simulink model "two_segment_model"  (R2024b)
settings: Solver=VariableStepAuto  StartTime=0.0  StopTime=0.64  MaxStep=0.001  RelTol=1e-6
values from neighbouring files (symbols this model uses):
  attack_angle = 90    [params.m]
  c = log(0.05)    [params.m]
  d = 0.04    [params.m]
  delP = 0.015    [params.m]
  e_ref_see = 0.04    [params.m]
  F_max = 22000    [params.m]
  g = 9.81    [params.m]
  G = 1.84/F_max    (= 8.36363636364e-05)    [params.m]
  K = 5    [params.m]
  l_f = 0.99    [params.m]
  l_off = 0.08    [params.m]
  l_opt = 0.1    [params.m]
  l_ref_mtc = 0.5    [params.m]
  l_rest = 0.4    [params.m]
  l_s = 0.5    [params.m]
  m = 80    [params.m]
  N = 1.5    [params.m]
  phi_initial = 2*rad2deg(atan(l_f/(2*sqrt(l_s^2 - l_f^2/4))))    [params.m]
  phi_ref_mtc = 110    [params.m]
  stim0 = 0.145    [params.m]
  tau = 0.01    [params.m]
  v_max = 12*l_opt    (= 1.2)    [params.m]
  w = 0.4    [params.m]
libraries: simulink_extras x1
settings Model: Creator=athar  LastModifiedBy=athar

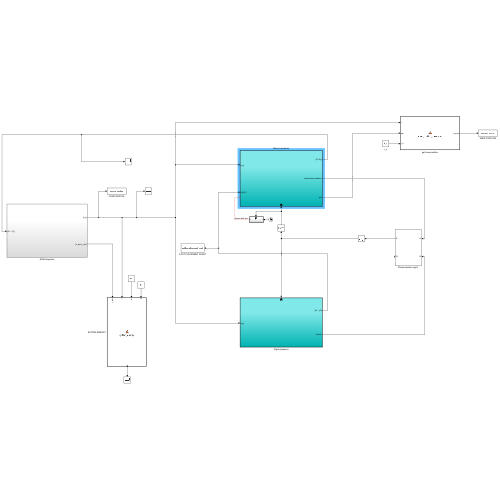
[thumbnail: Simulink's stored preview of the top-level diagram]
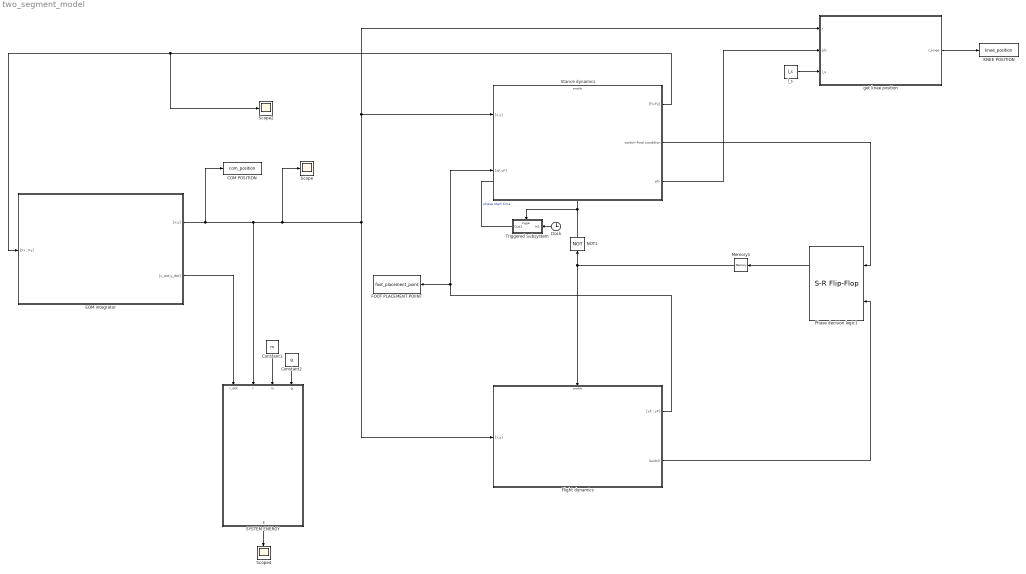
== system two_segment_model ==
  COM POSITION : ToWorkspace  VariableName=com_position  SampleTime=-1
      settings: Save2DSignal=2-D array (concatenate along first dimension)
  Clock : Clock
  Constant1 : Constant  Value=m
  Constant2 : Constant  Value=g
  EOM integrator : Subsystem
  FOOT PLACEMENT POIINT : ToWorkspace  VariableName=foot_placement_point  SampleTime=-1
      settings: Save2DSignal=2-D array (concatenate along first dimension)
  Flight dynamics : Subsystem
  KNEE POSITION : ToWorkspace  VariableName=knee_position  SampleTime=-1
      settings: Save2DSignal=2-D array (concatenate along first dimension)
  Memory1 : Memory  InitialCondition=1
  NOT1 : Logic  Operator=NOT  AllPortsSameDT=off  OutDataTypeStr=boolean
  Phase decision logic1 : simulink_extras/Flip Flops/S-R Flip-Flop  initial_condition=1
  SYSTEM ENERGY : MATLAB Function  TreatAsAtomicUnit=on
  Scope : Scope
  Scope2 : Scope
  Scope4 : Scope
  Stance dynamics : Subsystem
  Triggered Subsystem : Subsystem  TreatAsAtomicUnit=on
  get knee position : MATLAB Function  TreatAsAtomicUnit=on
  l_s : Constant  Value=l_s
  wires:
  Flight dynamics/1("[xF ; yF]") -> Stance dynamics/2("[xF,yF]"), FOOT PLACEMENT POIINT/1
  Stance dynamics/1("[Fx;Fy]") -> Scope2/1, EOM integrator/1("[Fx ; Fy]")
  Memory1/1 -> NOT1/1, Flight dynamics/Enable
  Flight dynamics/2(Switch) -> Phase decision logic1/2
  Phase decision logic1/1 -> Memory1/1
  NOT1/1 -> Triggered Subsystem/Trigger, Stance dynamics/Enable
  Stance dynamics/2(switch-final condition) -> Phase decision logic1/1
  EOM integrator/2("[x_dot;y_dot]") -> SYSTEM ENERGY/1(r_dot)
  Constant1/1 -> SYSTEM ENERGY/3(m)
  Constant2/1 -> SYSTEM ENERGY/4(g)
  SYSTEM ENERGY/1(E) -> Scope4/1
  Clock/1 -> Triggered Subsystem/1(In1)
  Triggered Subsystem/1(Out1) -> ?  "phase start time"
  EOM integrator/1("[x;y]") -> COM POSITION/1, SYSTEM ENERGY/2(r), Scope/1, Flight dynamics/1("[x;y]"), get knee position/1(r), Stance dynamics/1("[x,y]")
  Stance dynamics/3(phi) -> get knee position/2(phi)
  l_s/1 -> get knee position/3(l_s)
  get knee position/1(r_knee) -> KNEE POSITION/1

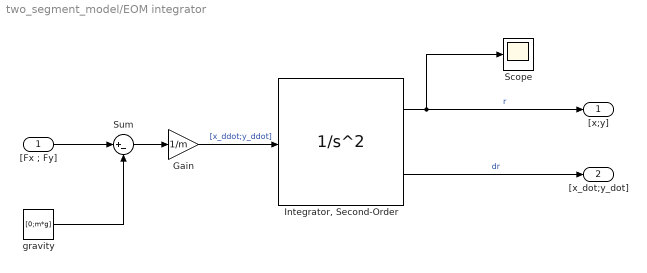
== system two_segment_model/EOM integrator ==
  "[Fx ; Fy]" : Inport
  Gain : Gain  Gain=1/m
  "Integrator, Second-Order" : SecondOrderIntegrator  ICX=r0  ICDXDT=r_dot0
  Scope : Scope
  Sum : Sum  Inputs=|+-
  gravity : Constant  Value=[0;m*g]
  "[x;y]" : Outport
  "[x_dot;y_dot]" : Outport  Port=2
  wires:
  "Integrator, Second-Order"/2 -> "[x_dot;y_dot]"/1  "dr"
  "Integrator, Second-Order"/1 -> Scope/1, "[x;y]"/1  "r"
  "[Fx ; Fy]"/1 -> Sum/1
  Sum/1 -> Gain/1
  gravity/1 -> Sum/2
  Gain/1 -> "Integrator, Second-Order"/1  "[x_ddot;y_ddot]"

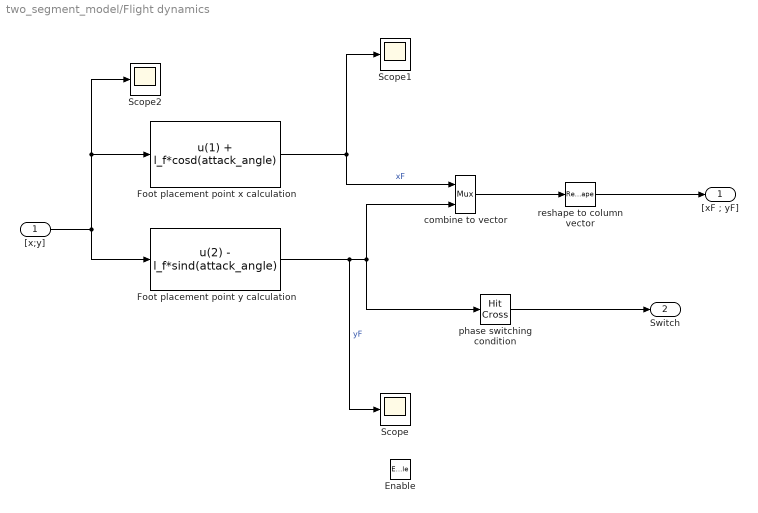
== system two_segment_model/Flight dynamics ==
  "[x;y]" : Inport
  Enable : EnablePort  StatesWhenEnabling=reset
  Foot placement point x calculation : Fcn  Expr=u(1) + l_f*cosd(attack_angle)
  Foot placement point y calculation : Fcn  Expr=u(2) - l_f*sind(attack_angle)
  Scope : Scope
  Scope1 : Scope
  Scope2 : Scope
  combine to vector : Mux  Inputs=2
  phase switching condition : HitCross  HitCrossingOffset=yG  HitCrossingDirection=falling
  reshape to column vector : Reshape  OutputDimensionality=Column vector (2-D)
  "[xF ; yF]" : Outport  InitialOutput=[0;0]
  Switch : Outport  Port=2  OutputWhenDisabled=reset  InitialOutput=0
  wires:
  "[x;y]"/1 -> Foot placement point y calculation/1, Scope2/1, Foot placement point x calculation/1
  Foot placement point y calculation/1 -> Scope/1, combine to vector/2, phase switching condition/1  "yF"
  Foot placement point x calculation/1 -> Scope1/1, combine to vector/1  "xF"
  combine to vector/1 -> reshape to column vector/1
  phase switching condition/1 -> Switch/1
  reshape to column vector/1 -> "[xF ; yF]"/1

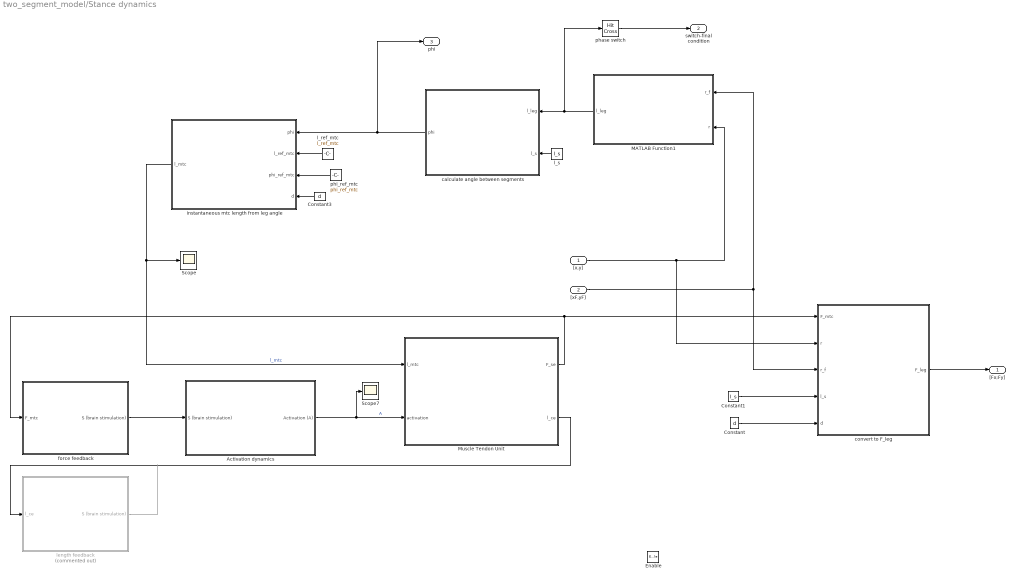
== system two_segment_model/Stance dynamics ==
  "[x,y]" : Inport
  "[xF,yF]" : Inport  Port=2
  Enable : EnablePort  StatesWhenEnabling=reset
  Activation dynamics : Subsystem
  Constant : Constant  Value=d
  Constant1 : Constant  Value=l_s
  Constant3 : Constant  Value=d
  MATLAB Function1 : MATLAB Function  TreatAsAtomicUnit=on
  Muscle Tendon Unit : Subsystem
  Scope : Scope
  Scope7 : Scope
  calculate angle between segments : MATLAB Function  TreatAsAtomicUnit=on
  convert to F_leg : MATLAB Function  TreatAsAtomicUnit=on
  force feedback : Subsystem
  instantaneous mtc length from leg angle : MATLAB Function  TreatAsAtomicUnit=on
  l_ref_mtc : Constant  Value=l_ref_mtc
  l_s : Constant  Value=l_s
  length feedback : Subsystem  Commented=on
  phase switch : HitCross  HitCrossingOffset=l_f  HitCrossingDirection=rising
  phi_ref_mtc : Constant  Value=phi_ref_mtc
  "[Fx;Fy]" : Outport  OutputWhenDisabled=reset  InitialOutput=[0;0]
  switch-final condition : Outport  Port=2  OutputWhenDisabled=reset  InitialOutput=0
  phi : Outport  Port=3  InitialOutput=phi_initial
  wires:
  "[xF,yF]"/1 -> MATLAB Function1/1(r_f), convert to F_leg/3(r_f)
  convert to F_leg/1(F_leg) -> "[Fx;Fy]"/1
  instantaneous mtc length from leg angle/1(l_mtc) -> Scope/1, Muscle Tendon Unit/1(l_mtc)  "l_mtc"
  l_ref_mtc/1 -> instantaneous mtc length from leg angle/2(l_ref_mtc)
  "[x,y]"/1 -> MATLAB Function1/2(r), convert to F_leg/2(r)
  Activation dynamics/1(Activation (A)) -> Scope7/1, Muscle Tendon Unit/2(activation)  "A"
  phi_ref_mtc/1 -> instantaneous mtc length from leg angle/3(phi_ref_mtc)
  Muscle Tendon Unit/1(F_se) -> force feedback/1(F_mtc), convert to F_leg/1(F_mtc)
  Constant/1 -> convert to F_leg/5(d)
  Constant1/1 -> convert to F_leg/4(l_s)
  l_s/1 -> calculate angle between segments/2(l_s)
  calculate angle between segments/1(phi) -> phi/1, instantaneous mtc length from leg angle/1(phi)
  Constant3/1 -> instantaneous mtc length from leg angle/4(d)
  MATLAB Function1/1(l_leg) -> phase switch/1, calculate angle between segments/1(l_leg)
  phase switch/1 -> switch-final condition/1
  Muscle Tendon Unit/2(l_ce) -> length feedback/1(l_ce)
  length feedback/1(S (brain stimulation)) -> ?
  force feedback/1(S (brain stimulation)) -> Activation dynamics/1(S (brain stimulation))

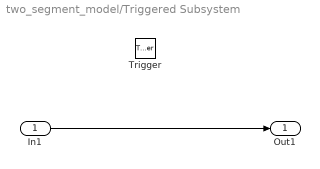
== system two_segment_model/Triggered Subsystem ==
  In1 : Inport
  Trigger : TriggerPort  VariantControl=(inherit)
  Out1 : Outport
  wires:
  In1/1 -> Out1/1

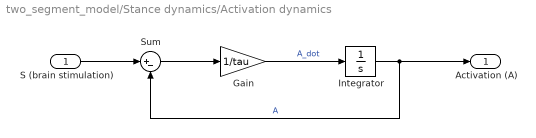
== system two_segment_model/Stance dynamics/Activation dynamics ==
  S (brain stimulation) : Inport
  Gain : Gain  Gain=1/tau
  Integrator : Integrator  InitialCondition=0.001
  Sum : Sum  Inputs=|+-
  Activation (A) : Outport
  wires:
  S (brain stimulation)/1 -> Sum/1
  Sum/1 -> Gain/1
  Gain/1 -> Integrator/1  "A_dot"
  Integrator/1 -> Sum/2, Activation (A)/1  "A"

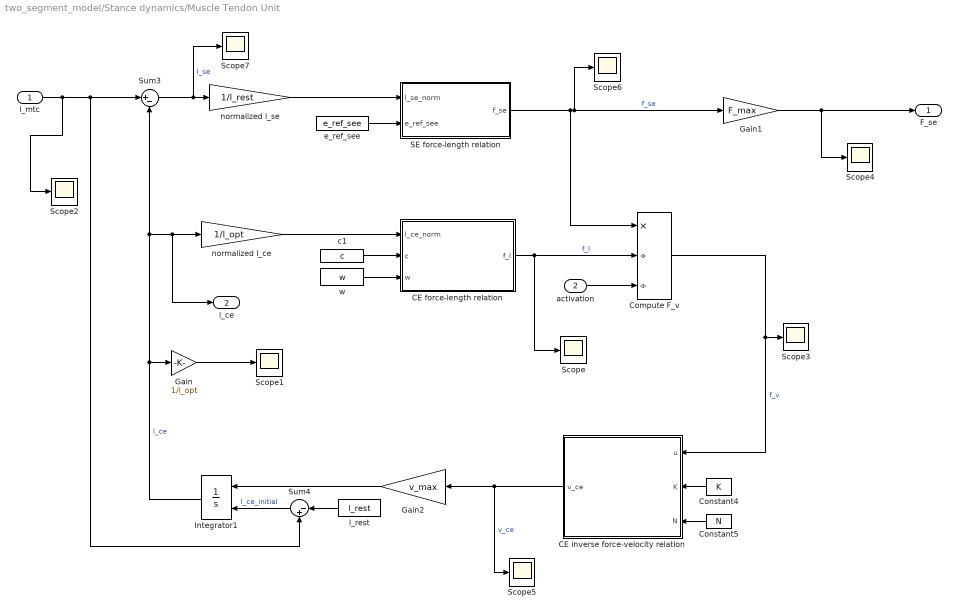
== system two_segment_model/Stance dynamics/Muscle Tendon Unit ==
  l_mtc : Inport
  activation : Inport  Port=2
  CE force-length relation : MATLAB Function  TreatAsAtomicUnit=on
  CE inverse force-velocity relation : MATLAB Function  TreatAsAtomicUnit=on
  Compute F_v : Product  Inputs=*//
  Constant4 : Constant  Value=K
  Constant5 : Constant  Value=N
  Gain : Gain  Gain=1/l_opt
  Gain1 : Gain  Gain=F_max
  Gain2 : Gain  Gain=v_max
  Integrator1 : Integrator  InitialConditionSource=external
  SE force-length relation : MATLAB Function  TreatAsAtomicUnit=on
  Scope{,1..7} (8 alike) : Scope
  Sum3 : Sum  Inputs=|+-
  Sum4 : Sum  Inputs=|-+
  c1 : Constant  Value=c
  e_ref_see : Constant  Value=e_ref_see
  l_rest : Constant  Value=l_rest
  normalized l_ce : Gain  Gain=1/l_opt
  normalized l_se : Gain  Gain=1/l_rest
  w : Constant  Value=w
  F_se : Outport
  l_ce : Outport  Port=2
  wires:
  SE force-length relation/1(f_se) -> Compute F_v/1, Gain1/1, Scope6/1  "f_se"
  activation/1 -> Compute F_v/3
  Integrator1/1 -> Gain/1, l_ce/1, normalized l_ce/1, Sum3/2  "l_ce"
  c1/1 -> CE force-length relation/2(c)
  normalized l_ce/1 -> CE force-length relation/1(l_ce_norm)
  CE inverse force-velocity relation/1(v_ce) -> Scope5/1, Gain2/1  "v_ce"
  Compute F_v/1 -> Scope3/1, CE inverse force-velocity relation/1(u)  "f_v"
  normalized l_se/1 -> SE force-length relation/1(l_se_norm)
  Constant5/1 -> CE inverse force-velocity relation/3(N)
  Gain2/1 -> Integrator1/1
  CE force-length relation/1(f_l) -> Scope/1, Compute F_v/2  "f_l"
  Sum4/1 -> Integrator1/2  "l_ce_initial"
  Sum3/1 -> Scope7/1, normalized l_se/1  "l_se"
  Gain1/1 -> Scope4/1, F_se/1
  l_rest/1 -> Sum4/1
  Constant4/1 -> CE inverse force-velocity relation/2(K)
  e_ref_see/1 -> SE force-length relation/2(e_ref_see)
  w/1 -> CE force-length relation/3(w)
  l_mtc/1 -> Scope2/1, Sum4/2, Sum3/1
  Gain/1 -> Scope1/1

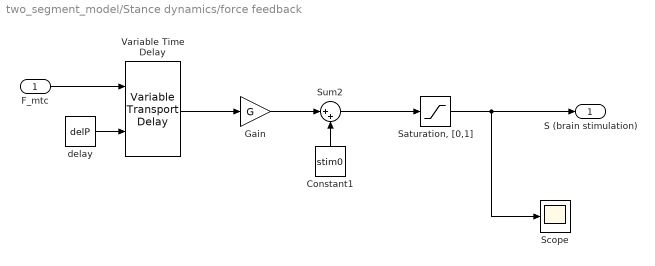
== system two_segment_model/Stance dynamics/force feedback ==
  F_mtc : Inport
  Constant1 : Constant  Value=stim0
  Gain : Gain  Gain=G
  "Saturation, [0,1]" : Saturate  UpperLimit=1  LowerLimit=0
  Scope : Scope
  Sum2 : Sum  Inputs=|++
  Variable Time Delay : VariableTransportDelay  MaximumDelay=10  MaximumPoints=1900000
  delay : Constant  Value=delP
  S (brain stimulation) : Outport
  wires:
  Constant1/1 -> Sum2/2
  "Saturation, [0,1]"/1 -> Scope/1, S (brain stimulation)/1
  Sum2/1 -> "Saturation, [0,1]"/1
  delay/1 -> Variable Time Delay/2
  Variable Time Delay/1 -> Gain/1
  F_mtc/1 -> Variable Time Delay/1
  Gain/1 -> Sum2/1

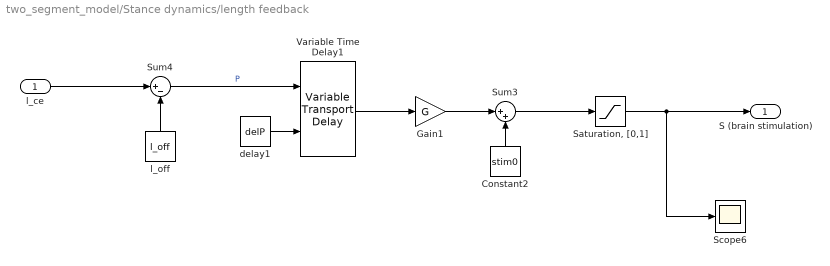
== system two_segment_model/Stance dynamics/length feedback ==
  l_ce : Inport
  Constant2 : Constant  Value=stim0
  Gain1 : Gain  Gain=G
  "Saturation, [0,1]" : Saturate  UpperLimit=1  LowerLimit=0
  Scope6 : Scope
  Sum3 : Sum  Inputs=|++
  Sum4 : Sum  Inputs=|+-
  Variable Time Delay1 : VariableTransportDelay  MaximumDelay=10  MaximumPoints=1900000
  delay1 : Constant  Value=delP
  l_off : Constant  Value=l_off
  S (brain stimulation) : Outport
  wires:
  Gain1/1 -> Sum3/1
  delay1/1 -> Variable Time Delay1/2
  Constant2/1 -> Sum3/2
  "Saturation, [0,1]"/1 -> Scope6/1, S (brain stimulation)/1
  Sum3/1 -> "Saturation, [0,1]"/1
  Variable Time Delay1/1 -> Gain1/1
  l_off/1 -> Sum4/2
  l_ce/1 -> Sum4/1
  Sum4/1 -> Variable Time Delay1/1  "P"

== matlab function two_segment_model/Stance dynamics/convert to F_leg ==
  data: F_mtc input; r input; r_f input; F_leg output; l_s input; d input
function F_leg = F_mtc_to_F_leg(F_mtc,r,r_f,l_s,d)

x = r(1); % Position of com
y = r(2);

x_f = r_f(1); % Position of foot
y_f = r_f(2);

l_leg = sqrt((x - x_f)^2 + (y - y_f)^2);

F_leg_magnitude = F_mtc*(d/sqrt(l_s^2 - l_leg^2/4)); % this is the magnitude, direction is along leg axis

F_leg_direction = (1/l_leg)*[x-x_f ; y-y_f];

F_leg = F_leg_magnitude*F_leg_direction;

end

== matlab function two_segment_model/Stance dynamics/calculate angle between segments ==
  data: l_leg input; phi output; l_s input
function phi = joint_angle_calculator(l_leg, l_s)

phi = 2*rad2deg(atan(l_leg/(2*(sqrt(l_s^2 - l_leg^2/4)))));  % Converts radians to degrees

end

== matlab function two_segment_model/Stance dynamics/instantaneous mtc length from leg angle ==
  data: phi input; l_mtc output; l_ref_mtc input; phi_ref_mtc input; d input
function l_mtc = l_mtc_calculator(phi, l_ref_mtc, phi_ref_mtc, d)

l_mtc = l_ref_mtc - d*deg2rad(phi - phi_ref_mtc);

end

== matlab function two_segment_model/Stance dynamics/MATLAB Function1 ==
  data: r_f input; r input; l_leg output
function l_leg = leg_length_calculator(r_f, r)

x = r(1); % Position of com
y = r(2);

x_f = r_f(1); % Position of foot
y_f = r_f(2);

l_leg = sqrt((x - x_f)^2 + (y - y_f)^2);

== matlab function two_segment_model/Stance dynamics/Muscle Tendon Unit/CE force-length relation ==
  data: l_ce_norm input; f_l output; c input; w input
function f_l = f_l(l_ce_norm, c , w)

    f_l = exp(c * (abs((l_ce_norm - 1) / w)^3));

end

== matlab function two_segment_model/SYSTEM ENERGY ==
  data: r_dot input; r input; m input; E output; g input
function E= system_energy(r_dot , r , m , g)

x = r(1); % Position of com
y = r(2);

v_x = r_dot(1); % Position of foot
v_y = r_dot(2);

E = 0.5*m*(v_x^2 + v_y^2) + m*g*y;

end

== matlab function two_segment_model/get knee position ==
  data: r input; r_knee output; phi input; l_s input
function r_knee = knee_position_calculator(r , phi, l_s)

x = r(1);
y = r(2);

x_knee = x + l_s*cosd(phi/2);
y_knee = y - l_s*sind(phi/2);

r_knee = [x_knee ; y_knee];

== matlab function two_segment_model/Stance dynamics/Muscle Tendon Unit/CE inverse force-velocity relation ==
  data: u input; v_ce output; K input; N input
function v_ce = f_v_inverse(u, K, N)
  
    if u < 1
        v_ce = (u - 1)/(1 + K * u);
    
    elseif (1 <= u) && (u < N)
        v_ce = (1 - u) / ((1 - N) + 7.56 * K * (u - N));
    
    elseif u >= N
        v_ce = 1;
    
    else 
        v_ce = 0;
    end
    
end

== matlab function two_segment_model/Stance dynamics/Muscle Tendon Unit/SE force-length relation ==
  data: l_se_norm input; f_se output; e_ref_see input
function f_se = f_se(l_se_norm, e_ref_see)

e = l_se_norm - 1;

if e > 0
    f_se = (e / e_ref_see)^2;
else
    f_se = 0;
end
